simulink model "p4_simulink"  (R2020b)
settings: Solver=VariableStepAuto  StartTime=0.0  StopTime=15  MaxStep=0.001  RelTol=1e-4
values from neighbouring files (symbols this model uses):
  parede = 25    [p4.m]
libraries: simulink x2
settings Model: Creator=35193  LastModifiedBy=35193
settings SolverCC: ZeroCrossAlgorithm=Adaptive
settings DebuggingCC: IgnoredZcDiagnostic=none

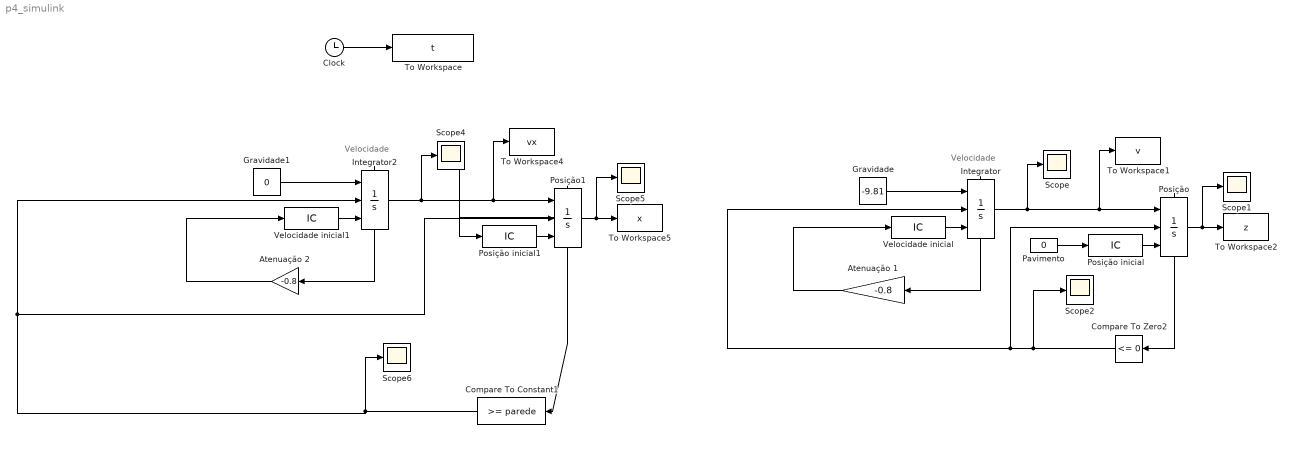
== system p4_simulink ==
  note: Velocidade
  note: Velocidade
  Atenuação 1 : Gain  Gain=-0.8
  Atenuação 2 : Gain  Gain=-0.8
  Clock : Clock
  Compare To Constant1 : simulink/Logic and Bit Operations/Compare To Constant  relop=>=  const=parede  OutDataTypeStr=boolean
  Compare To Zero2 : simulink/Logic and Bit Operations/Compare To Zero  relop=<=  OutDataTypeStr=boolean
  Gravidade : Constant  Value=-9.81
  Gravidade1 : Constant  Value=0
  Integrator : Integrator  ExternalReset=rising  InitialConditionSource=external  ShowStatePort=on
  Integrator2 : Integrator  ExternalReset=rising  InitialConditionSource=external  ShowStatePort=on
  Pavimento : Constant  Value=0
  Posição : Integrator  ExternalReset=rising  InitialConditionSource=external  LimitOutput=on  LowerSaturationLimit=0  ShowStatePort=on
  Posição inicial : InitialCondition  Value=10
  Posição inicial1 : InitialCondition  Value=0
  Posição1 : Integrator  ExternalReset=rising  InitialConditionSource=external  LimitOutput=on  ShowStatePort=on
  Scope{,1..2,4..6} (6 alike) : Scope
  To Workspace : ToWorkspace  VariableName=t  SampleTime=-1
      settings: Save2DSignal=2-D array (concatenate along first dimension)
  To Workspace1 : ToWorkspace  VariableName=v  SampleTime=-1
      settings: Save2DSignal=2-D array (concatenate along first dimension)
  To Workspace2 : ToWorkspace  VariableName=z  SampleTime=-1
      settings: Save2DSignal=2-D array (concatenate along first dimension)
  To Workspace4 : ToWorkspace  VariableName=vx  SampleTime=-1
      settings: Save2DSignal=2-D array (concatenate along first dimension)
  To Workspace5 : ToWorkspace  VariableName=x  SampleTime=-1
      settings: Save2DSignal=2-D array (concatenate along first dimension)
  Velocidade inicial : InitialCondition  Value=0
  Velocidade inicial1 : InitialCondition  Value=7
  wires:
  Clock/1 -> To Workspace/1
  Gravidade/1 -> Integrator/1
  Integrator/1 -> Posição/1, To Workspace1/1, Scope/1
  Compare To Zero2/1 -> Integrator/2, Posição/2, Scope2/1
  Posição inicial/1 -> Posição/3
  Pavimento/1 -> Posição inicial/1
  Velocidade inicial/1 -> Integrator/3
  Posição/1 -> Scope1/1, To Workspace2/1
  Integrator/State -> Atenuação 1/1
  Atenuação 1/1 -> Velocidade inicial/1
  Atenuação 2/1 -> Velocidade inicial1/1
  Posição1/State -> Posição inicial1/1, Compare To Constant1/1
  Posição inicial1/1 -> Posição1/3
  Posição1/1 -> Scope5/1, To Workspace5/1
  Velocidade inicial1/1 -> Integrator2/3
  Integrator2/State -> Atenuação 2/1
  Gravidade1/1 -> Integrator2/1
  Integrator2/1 -> Posição1/1, To Workspace4/1, Scope4/1
  Compare To Constant1/1 -> Integrator2/2, Posição1/2, Scope6/1
  Posição/State -> Compare To Zero2/1
